simulink model "cordicModelComposer"  (R2021a)
settings: Solver=VariableStepAuto  StartTime=0.0  StopTime=50  RelTol=1e-3
undefined symbols (not defined in the file or in its folder): A, N
libraries: hdlBasic x26, hdlDSPIP x2, xbsIndex_r4 x1, JTAGRuntimeCosim_r4 x1
settings Model: Creator=Heather  LastModifiedBy=kv25
settings DebuggingCC: UnconnectedInputMsg=none  UnconnectedOutputMsg=none  UnconnectedLineMsg=none
settings ModelReferenceCC: EnableRefExpFcnMdlSchedulingChecks=off
settings RTWCC: Description=Generic Real-Time Target  DLArmComputeVersion=20.02.1

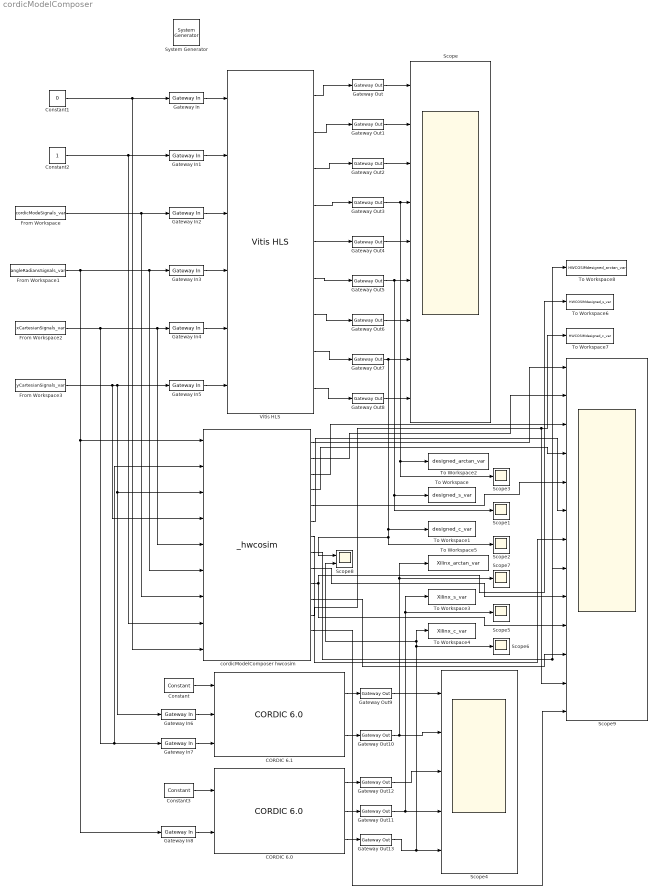
== system cordicModelComposer ==
  " System Generator" : xbsIndex_r4/ System Generator  Tag=genX  xilinxfamily=zynq  part=xc7z020  speed=-1  package=clg484  synthesis_tool=Vivado  clock_wrapper=Clock Enables  directory=./netlist369  proj_type=Vivado  Synth_file=Vivado Synthesis Defaults  Impl_file=Vivado Implementation Defaults  testbench=off  simulink_period=1  sysclk_period=10  dcm_input_clock_period=10  incr_netlist=off  trim_vbits=Everywhere in SubSystem  dbl_ovrd=According to Block Masks  core_generation=According to Block Masks  run_coregen=off  deprecated_control=off  eval_field=0  block_type=sysgen
  CORDIC 6.0 : hdlDSPIP/CORDIC 6.0   functional_selection=Sin_and_Cos  architectural_configuration=Parallel  pipelining_mode=Maximum  data_format=SignedFraction  phase_format=Radians  input_width=16  output_width=16  round_mode=Truncate  iterations=20  precision=0  compensation_scaling=No_Scale_Compensation  coarse_rotation=on  aclken=off  aresetn=off  out_tready=off  cartesian_has_tuser=off  cartesian_has_tlast=off  cartesian_tuser_width=1  phase_has_tuser=off  phase_has_tlast=off  phase_tuser_width=1  out_tlast_behv=Null  flow_control=NonBlocking  optimize_goal=Resources  trim_axipin_name=on  simulation_type=hybrid_sim  simulation_model=sysgen:cordic_v6_0  data_path_portlist={'s_axis_cartesian_tdata_imag', 's_axis_cartesian_tdata_real', 's_axis_phase_tdata_phase', 'm_axis_dout_tdata_imag', 'm_axis_dout_tdata_real', 'm_axis_dout_tdata_phase','m_axis_dout_tdata'}  ip_name=CORDIC  ip_version=6.0  dsptool_ready=true  ipcore_usecache=true  ipcore_useipmodelcache=true  wrapper_available=true  port_translation_map={ 'aclken' => 'en', 'aresetn' => 'rst' }  XmcBlockStatus=1  maskContainerNames=group15  block_type=cordic_v6_0  block_config=sysgen:rodinimport_config  block_width=800
  CORDIC 6.1 : hdlDSPIP/CORDIC 6.0   functional_selection=Arc_Tan  architectural_configuration=Parallel  pipelining_mode=Maximum  data_format=SignedFraction  phase_format=Radians  input_width=16  output_width=16  round_mode=Truncate  iterations=0  precision=0  compensation_scaling=No_Scale_Compensation  coarse_rotation=on  aclken=off  aresetn=off  out_tready=off  cartesian_has_tuser=off  cartesian_has_tlast=off  cartesian_tuser_width=1  phase_has_tuser=off  phase_has_tlast=off  phase_tuser_width=1  out_tlast_behv=Null  flow_control=NonBlocking  optimize_goal=Resources  trim_axipin_name=on  simulation_type=hybrid_sim  simulation_model=sysgen:cordic_v6_0  data_path_portlist={'s_axis_cartesian_tdata_imag', 's_axis_cartesian_tdata_real', 's_axis_phase_tdata_phase', 'm_axis_dout_tdata_imag', 'm_axis_dout_tdata_real', 'm_axis_dout_tdata_phase','m_axis_dout_tdata'}  ip_name=CORDIC  ip_version=6.0  dsptool_ready=true  ipcore_usecache=true  ipcore_useipmodelcache=true  wrapper_available=true  port_translation_map={ 'aclken' => 'en', 'aresetn' => 'rst' }  XmcBlockStatus=1  maskContainerNames=group15  block_type=cordic_v6_0  block_config=sysgen:rodinimport_config  block_width=800
  Constant : hdlBasic/Constant  const=1.0  gui_display_data_type=Boolean  arith_type=Boolean  n_bits=16  bin_pt=14  preci_type=Single  exp_width=8  frac_width=24  explicit_period=off  period=1  XmcBlockStatus=1  maskContainerNames=tabcontainer1  block_type=constant  block_config=sysgen:Constant_config
  Constant1 : Constant  Value=0
  Constant2 : Constant
  Constant3 : hdlBasic/Constant  const=1.0  gui_display_data_type=Boolean  arith_type=Boolean  n_bits=16  bin_pt=14  preci_type=Single  exp_width=8  frac_width=24  explicit_period=off  period=1  XmcBlockStatus=1  maskContainerNames=tabcontainer1  block_type=constant  block_config=sysgen:Constant_config
  From Workspace : FromWorkspace  VariableName=cordicModeSignals_var
  From Workspace1 : FromWorkspace  VariableName=angleRadiansSignals_var
  From Workspace2 : FromWorkspace  VariableName=xCartesianSignals_var
  From Workspace3 : FromWorkspace  VariableName=yCartesianSignals_var
  Gateway In : hdlBasic/Gateway In  gui_display_data_type=Boolean  arith_type=Boolean  n_bits=16  bin_pt=14  preci_type=Single  exp_width=8  frac_width=24  rows=1  columns=1  quantization="Round  (unbiased: +/- Inf)"  overflow=Saturate  period=1  UseAsADC=off  ADCChannel='1'  interface=None  automatic_assignment=on  address_offset=hex2dec('00')  intf_name=''  intf_description=''  default_value=0  timing_constraint=None  locs_specified=off  LOCs={}  io_standard={}  inherit_from_input=off  hdl_port=on  XmcBlockStatus=1  maskContainerNames=group4  block_type=gatewayin  block_config=sysgen:gateway_in_config  block_width_w=590  block_height_w=620  block_width=640  block_height=850
  Gateway In1 : hdlBasic/Gateway In  gui_display_data_type=Boolean  arith_type=Boolean  n_bits=16  bin_pt=3  preci_type=Single  exp_width=8  frac_width=24  rows=1  columns=1  quantization="Round  (unbiased: +/- Inf)"  overflow=Saturate  period=1  UseAsADC=off  ADCChannel='1'  interface=None  automatic_assignment=on  address_offset=hex2dec('00')  intf_name=''  intf_description=''  default_value=0  timing_constraint=None  locs_specified=off  LOCs={}  io_standard={}  inherit_from_input=off  hdl_port=on  XmcBlockStatus=1  maskContainerNames=group4  block_type=gatewayin  block_config=sysgen:gateway_in_config  block_width_w=590  block_height_w=620  block_width=640  block_height=850
  Gateway In2 : hdlBasic/Gateway In  gui_display_data_type=Boolean  arith_type=Boolean  n_bits=16  bin_pt=3  preci_type=Single  exp_width=8  frac_width=24  rows=1  columns=1  quantization="Round  (unbiased: +/- Inf)"  overflow=Saturate  period=1  UseAsADC=off  ADCChannel='1'  interface=None  automatic_assignment=on  address_offset=hex2dec('00')  intf_name=''  intf_description=''  default_value=0  timing_constraint=None  locs_specified=off  LOCs={}  io_standard={}  inherit_from_input=off  hdl_port=on  XmcBlockStatus=1  maskContainerNames=group4  block_type=gatewayin  block_config=sysgen:gateway_in_config  block_width_w=590  block_height_w=620  block_width=640  block_height=850
  Gateway In{3..5,8} (4 alike) : hdlBasic/Gateway In  gui_display_data_type=Fixed-point  arith_type=Signed (2's comp)  n_bits=16  bin_pt=13  preci_type=Single  exp_width=8  frac_width=24  rows=1  columns=1  quantization="Round  (unbiased: +/- Inf)"  overflow=Saturate  period=1  UseAsADC=off  ADCChannel='1'  interface=None  automatic_assignment=on  address_offset=hex2dec('00')  intf_name=''  intf_description=''  default_value=0  timing_constraint=None  locs_specified=off  LOCs={}  io_standard={}  inherit_from_input=off  hdl_port=on  XmcBlockStatus=1  maskContainerNames=group4  block_type=gatewayin  block_config=sysgen:gateway_in_config  block_width_w=590  block_height_w=620  block_width=640  block_height=850
  Gateway In6 : hdlBasic/Gateway In  gui_display_data_type=Fixed-point  arith_type=Signed (2's comp)  n_bits=16  bin_pt=14  preci_type=Single  exp_width=8  frac_width=24  rows=1  columns=1  quantization="Round  (unbiased: +/- Inf)"  overflow=Saturate  period=1  UseAsADC=off  ADCChannel='1'  interface=None  automatic_assignment=on  address_offset=hex2dec('00')  intf_name=''  intf_description=''  default_value=0  timing_constraint=None  locs_specified=off  LOCs={}  io_standard={}  inherit_from_input=off  hdl_port=on  XmcBlockStatus=1  maskContainerNames=group4  block_type=gatewayin  block_config=sysgen:gateway_in_config  block_width_w=590  block_height_w=620  block_width=640  block_height=850
  Gateway In7 : hdlBasic/Gateway In  gui_display_data_type=Fixed-point  arith_type=Signed (2's comp)  n_bits=16  bin_pt=14  preci_type=Single  exp_width=8  frac_width=24  rows=1  columns=1  quantization="Round  (unbiased: +/- Inf)"  overflow=Saturate  period=1  UseAsADC=off  ADCChannel='1'  interface=None  automatic_assignment=on  address_offset=hex2dec('00')  intf_name=''  intf_description=''  default_value=0  timing_constraint=None  locs_specified=off  LOCs={}  io_standard={}  inherit_from_input=off  hdl_port=on  XmcBlockStatus=1  maskContainerNames=group4  block_type=gatewayin  block_config=sysgen:gateway_in_config  block_width_w=590  block_height_w=620  block_width=640  block_height=850
  Gateway Out{,1..13} (14 alike) : hdlBasic/Gateway Out  inherit_from_input=off  hdl_port=on  rows=1  columns=1  UseAsDAC=off  DACChannel='1'  interface=None  automatic_assignment=on  address_offset=hex2dec('00')  intf_name=''  intf_description=''  timing_constraint=None  locs_specified=off  LOCs={}  io_standard={}  XmcBlockStatus=1  maskContainerNames=group4  block_type=gatewayout  block_config=sysgen:gateway_out_config  block_width_w=590  block_height_w=620  block_width=620  block_height=750
  Scope : Scope  NumInputPorts=9
  Scope{1..3,5..7} (6 alike) : Scope
  Scope4 : Scope  NumInputPorts=5
  Scope8 : Scope  NumInputPorts=2
  Scope9 : Scope  NumInputPorts=13
  To Workspace : ToWorkspace  VariableName=designed_s_var  SaveFormat=Timeseries  SampleTime=-1
  To Workspace1 : ToWorkspace  VariableName=designed_c_var  SaveFormat=Timeseries  SampleTime=-1
  To Workspace2 : ToWorkspace  VariableName=designed_arctan_var  SaveFormat=Timeseries  SampleTime=-1
  To Workspace3 : ToWorkspace  VariableName=Xilinx_s_var  SaveFormat=Timeseries  SampleTime=-1
  To Workspace4 : ToWorkspace  VariableName=Xilinx_c_var  SaveFormat=Timeseries  SampleTime=-1
  To Workspace5 : ToWorkspace  VariableName=Xilinx_arctan_var  SaveFormat=Timeseries  SampleTime=-1
  To Workspace6 : ToWorkspace  VariableName=HWCOSIMdesigned_s_var  SaveFormat=Timeseries  SampleTime=-1
  To Workspace7 : ToWorkspace  VariableName=HWCOSIMdesigned_c_var  SaveFormat=Timeseries  SampleTime=-1
  To Workspace8 : ToWorkspace  VariableName=HWCOSIMdesigned_arctan_var  SaveFormat=Timeseries  SampleTime=-1
  Vitis HLS : hdlBasic/Vitis HLS  anytable='C:\ELEC522\venaik\Project4\Vitis_HLS\cordic\solution1'  fast_sim=on  display_datatype=off  rate_propagation_method=Simulink system period  model_file_path=''  latency=1  block_type=vitis_hls
      settings: infoedit=This block allows including C,C++ and SystemC source files in System Generator for DSP designs.
  cordicModelComposer hwcosim : JTAGRuntimeCosim_r4/_hwcosim  clkSrc=Single Stepped  hasCombinationalPath=on  bitfileName=C:\ELEC522\venaik\Project4\Vitis_MC\netlist369\cordicmodelcomposer.bit  skipConfig=off  dispPartInfo=off  useZynqReconfigScript=on  cable=Auto Detect  speed=N/A  cablePort=N/A  cableLocation=Local  shareCable=off  xmp=[]  software_settings=[]  design_xtable=|  binDir=[]  engineDll=JTAGCosimEngine.dll  cableWaitTime=10  bscanPos=-1  IRLengths=[]  useWaitBox=1  hasBufgmux=on  Scheme=Cosim  useCmdProc=1  hasProc=0  useImpact=0  printLogFile=0  userChain=2  XmcBlockStatus=0  maskContainerNames=tabcontainer1  block_type=jtagcosim  block_config=Sysgen:hwcosim_block_config
      | {
      |     'clkWrapper' => 'cordicmodelcomposer',
      |     'burstMode' => false,
      |     'burstFifoDepth' => '1024',
      |     'shared_memories' => {},
      |     'clocksGcd' => 1,
      |     'device' => {
      |       'family' => 'zynq',
      |       'part' => 'xc7z020',
      |       'package' => 'clg484',
      |       'speed' => '-1',
      |     },
      |     'ports' => {
      |       'gateway_in8' => {
      |         'direction' => 'in',
      |         'width' => 16,
      |         'name' => 'gateway_in8',
      |         'period' => 1,
      |         'icon_text' => 'Gateway In8',
      |         'type' => 'Fix_16_13',
      |         'arithmetic_type' => 'xlSigned',
      |         'dat_file' => 'cordicmodelcomposer_gateway_in8.dat',
      |         'bin_pt' => 13,
      |         'addr_offset' => 0,
      |         'bd_port_index' => 0,
      |       },
      |       'gateway_in7' => {
      |         'direction' => 'in',
      |         'width' => 16,
      |         'name' => 'gateway_in7',
      |         'period' => 1,
      |         'icon_text' => 'Gateway In7',
      |         'type' => 'Fix_16_14',
      |         'arithmetic_type' => 'xlSigned',
      |         'dat_file' => 'cordicmodelcomposer_gateway_in7.dat',
      |         'bin_pt' => 14,
      |         'addr_offset' => 4,
      |         'bd_port_index' => 1,
      |       },
      |       'gateway_in6' => {
      |         'direction' => 'in',
      |         'width' => 16,
      |         'name' => 'gateway_in6',
      |         'period' => 1,
      |         'icon_text' => 'Gateway In6',
      |         'type' => 'Fix_16_14',
      |         'arithmetic_type' => 'xlSigned',
      |         'dat_file' => 'cordicmodelcomposer_gateway_in6.dat',
      |         'bin_pt' => 14,
      |         'addr_offset' => 8,
      |         'bd_port_index' => 2,
      |       },
      |       'gateway_in5' => {
      |         'direction' => 'in',
      |         'width' => 16,
      |         'name' => 'gateway_in5',
      |         'period' => 1,
      |         'icon_text' => 'Gateway In5',
      |         'type' => 'Fix_16_13',
      |         'arithmetic_type' => 'xlSigned',
      |         'dat_file' => 'cordicmodelcomposer_gateway_in5.dat',
      |         'bin_pt' => 13,
      |         'addr_offset' => 12,
      |         'bd_port_index' => 3,
      |       },
      |       'gateway_in4' => {
      |         'direction' => 'in',
      |         'width' => 16,
      |         'name' => 'gateway_in4',
      |         'period' => 1,
      |         'icon_text' => 'Gateway In4',
      |         'type' => 'Fix_16_13',
      |         'arithmetic_type' => 'xlSigned',
      |         'dat_file' => 'cordicmodelcomposer_gateway_in4.dat',
      |         'bin_pt' => 13,
      |         'addr_offset' => 16,
      |         'bd_port_index' => 4,
      |       },
      |       'gateway_in3' => {
      |         'direction' => 'in',
      |         'width' => 16,
      |         'name' => 'gateway_in3',
      |         'period' => 1,
      |         'icon_text' => 'Gateway In3',
      |         'type' => 'Fix_16_13',
      |         'arithmetic_type' => 'xlSigned',
      |         'dat_file' => 'cordicmodelcomposer_gateway_in3.dat',
      |         'bin_pt' => 13,
      |         'addr_offset' => 20,
      |         'bd_port_index' => 5,
      |       },
      |       'gateway_in2' => {
      |         'direction' => 'in',
      |         'width' => 1,
      |         'name' => 'gateway_in2',
      |         'period' => 1,
      |         'icon_text' => 'Gateway In2',
      |         'type' => 'Bool',
      |         'arithmetic_type' => 'xlUnsigned',
      |         'dat_file' => 'cordicmodelcomposer_gateway_in2.dat',
      |         'bin_pt' => 0,
      |         'addr_offset' => 24,
      |         'bd_port_index' => 6,
      |       },
      |       'gateway_in1' => {
      |         'direction' => 'in',
      |         'width' => 1,
      |         'name' => 'gateway_in1',
      |         'period' => 1,
      |         'icon_text' => 'Gateway In1',
      |         'type' => 'Bool',
      |         'arithmetic_type' => 'xlUnsigned',
      |         'dat_file' => 'cordicmodelcomposer_gateway_in1.dat',
      |         'bin_pt' => 0,
      |         'addr_offset' => 28,
      |         'bd_port_index' => 7,
      |       },
      |       'gateway_in' => {
      |         'direction' => 'in',
      |         'width' => 1,
      |         'name' => 'gateway_in',
      |         'period' => 1,
      |         'icon_text' => 'Gateway In',
      |         'type' => 'Bool',
      |         'arithmetic_type' => 'xlUnsigned',
      |         'dat_file' => 'cordicmodelcomposer_gateway_in.dat',
      |         'bin_pt' => 0,
      |         'addr_offset' => 32,
      |         'bd_port_index' => 8,
      |       },
      |       'gateway_out' => {
      |         'direction' => 'out',
      |         'width' => 1,
      |         'name' => 'gateway_out',
      |         'period' => 1,
      |         'icon_text' => 'Gateway Out',
      |         'type' => 'Bool',
      |         'arithmetic_type' => 'xlUnsigned',
      |         'dat_file' => 'cordicmodelcomposer_gateway_out.dat',
      |         'bin_pt' => 0,
      |         'addr_offset' => 36,
      |         'bd_port_index' => 0,
      |       },
      |       'gateway_out1' => {
      |         'direction' => 'out',
      |         'width' => 1,
      |         'name' => 'gateway_out1',
      |         'period' => 1,
      |         'icon_text' => 'Gateway Out1',
      |         'type' => 'Bool',
      |         'arithmetic_type' => 'xlUnsigned',
      |         'dat_file' => 'cordicmodelcomposer_gateway_out1.dat',
      |         'bin_pt' => 0,
      |         'addr_offset' => 40,
      |         'bd_port_index' => 1,
      |       },
      |       'gateway_out10' => {
      |         'direction' => 'out',
      |         'width' => 16,
      |         'name' => 'gateway_out10',
      |         'period' => 1,
      |         'icon_text' => 'Gateway Out10',
      |         'type' => 'Fix_16_13',
      |         'arithmetic_type' => 'xlSigned',
      |         'dat_file' => 'cordicmodelcomposer_gateway_out10.dat',
      |         'bin_pt' => 13,
      |         'addr_offset' => 44,
      |         'bd_port_index' => 2,
      |       },
      |       'gateway_out11' => {
      |         'direction' => 'out',
      |         'width' => 16,
      |         'name' => 'gateway_out11',
      |         'period' => 1,
      |         'icon_text' => 'Gateway Out11',
      |         'type' => 'Fix_16_14',
      |         'arithmetic_type' => 'xlSigned',
      |         'dat_file' => 'cordicmodelcomposer_gateway_out11.dat',
      |         'bin_pt' => 14,
      |         'addr_offset' => 48,
      |         'bd_port_index' => 3,
      |       },
      |       'gateway_out12' => {
      |         'direction' => 'out',
      |         'width' => 1,
      |         'name' => 'gateway_out12',
      |         'period' => 1,
      |         'icon_text' => 'Gateway Out12',
      |         'type' => 'Bool',
      |         'arithmetic_type' => 'xlUnsigned',
      |         'dat_file' => 'cordicmodelcomposer_gateway_out12.dat',
      |         'bin_pt' => 0,
      |         'addr_offset' => 52,
      |         'bd_port_index' => 4,
      |       },
      |       'gateway_out13' => {
      |         'direction' => 'out',
      |         'width' => 16,
      |         'name' => 'gateway_out13',
      |         'period' => 1,
      |         'icon_text' => 'Gateway Out13',
      |         'type' => 'Fix_16_14',
      |         'arithmetic_type' => 'xlSigned',
      |         'dat_file' => 'cordicmodelcomposer_gateway_out13.dat',
      |         'bin_pt' => 14,
      |         'addr_offset' => 56,
      |         'bd_port_index' => 5,
      |       },
      |       'gateway_out2' => {
      |         'direction' => 'out',
      |         'width' => 1,
      |         'name' => 'gateway_out2',
      |         'period' => 1,
      |         'icon_text' => 'Gateway Out2',
      |         'type' => 'Bool',
      |         'arithmetic_type' => 'xlUnsigned',
      |         'dat_file' => 'cordicmodelcomposer_gateway_out2.dat',
      |         'bin_pt' => 0,
      |         'addr_offset' => 60,
      |         'bd_port_index' => 6,
      |       },
      |       'gateway_out3' => {
      |         'direction' => 'out',
      |         'width' => 16,
      |         'name' => 'gateway_out3',
      |         'period' => 1,
      |         'icon_text' => 'Gateway Out3',
      |         'type' => 'Fix_16_13',
      |         'arithmetic_type' => 'xlSigned',
      |         'dat_file' => 'cordicmodelcomposer_gateway_out3.dat',
      |         'bin_pt' => 13,
      |         'addr_offset' => 64,
      |         'bd_port_index' => 7,
      |       },
      |       'gateway_out4' => {
      |         'direction' => 'out',
      |         'width' => 1,
      |         'name' => 'gateway_out4',
      |         'period' => 1,
      |         'icon_text' => 'Gateway Out4',
      |         'type' => 'Bool',
      |         'arithmetic_type' => 'xlUnsigned',
      |         'dat_file' => 'cordicmodelcomposer_gateway_out4.dat',
      |         'bin_pt' => 0,
      |         'addr_offset' => 68,
      |         'bd_port_index' => 8,
      |       },
      |       'gateway_out5' => {
      |         'direction' => 'out',
      |         'width' => 16,
      |         'name' => 'gateway_out5',
      |         'period' => 1,
      |         'icon_text' => 'Gateway Out5',
      |         'type' => 'Fix_16_13',
      |         'arithmetic_type' => 'xlSigned',
      |         'dat_file' => 'cordicmodelcomposer_gateway_out5.dat',
      |         'bin_pt' => 13,
      |         'addr_offset' => 72,
      |         'bd_port_index' => 9,
      |       },
      |       'gateway_out6' => {
      |         'direction' => 'out',
      |         'width' => 1,
      |         'name' => 'gateway_out6',
      |         'period' => 1,
      |         'icon_text' => 'Gateway Out6',
      |         'type' => 'Bool',
      |         'arithmetic_type' => 'xlUnsigned',
      |         'dat_file' => 'cordicmodelcomposer_gateway_out6.dat',
      |         'bin_pt' => 0,
      |         'addr_offset' => 76,
      |         'bd_port_index' => 10,
      |       },
      |       'gateway_out7' => {
      |         'direction' => 'out',
      |         'width' => 16,
      |         'name' => 'gateway_out7',
      |         'period' => 1,
      |         'icon_text' => 'Gateway Out7',
      |         'type' => 'Fix_16_13',
      |         'arithmetic_type' => 'xlSigned',
      |         'dat_file' => 'cordicmodelcomposer_gateway_out7.dat',
      |         'bin_pt' => 13,
      |         'addr_offset' => 80,
      |         'bd_port_index' => 11,
      |       },
      |       'gateway_out8' => {
      |         'direction' => 'out',
      |         'width' => 1,
      |         'name' => 'gateway_out8',
      |         'period' => 1,
      |         'icon_text' => 'Gateway Out8',
      |         'type' => 'Bool',
      |         'arithmetic_type' => 'xlUnsigned',
      |         'dat_file' => 'cordicmodelcomposer_gateway_out8.dat',
      |         'bin_pt' => 0,
      |         'addr_offset' => 84,
      |         'bd_port_index' => 12,
      |       },
      |       'gateway_out9' => {
      |         'direction' => 'out',
      |         'width' => 1,
      |         'name' => 'gateway_out9',
      |         'period' => 1,
      |         'icon_text' => 'Gateway Out9',
      |         'type' => 'Bool',
      |         'arithmetic_type' => 'xlUnsigned',
      |         'dat_file' => 'cordicmodelcomposer_gateway_out9.dat',
      |         'bin_pt' => 0,
      |         'addr_offset' => 88,
      |         'bd_port_index' => 13,
      |       },
      |     },
      |   }
  wires:
  Constant2/1 -> cordicModelComposer hwcosim/8, Gateway In1/1
  Gateway In1/1 -> Vitis HLS/2
  Gateway In/1 -> Vitis HLS/1
  Constant1/1 -> cordicModelComposer hwcosim/9, Gateway In/1
  Vitis HLS/1 -> Gateway Out/1
  Vitis HLS/2 -> Gateway Out1/1
  Gateway Out/1 -> Scope/1
  Gateway Out1/1 -> Scope/2
  Gateway Out2/1 -> Scope/3
  Gateway Out4/1 -> Scope/5
  Gateway Out5/1 -> Scope/6, To Workspace/1, Scope1/1
  Gateway Out6/1 -> Scope/7
  Gateway Out7/1 -> Scope/8, Scope8/1, Scope2/1, To Workspace1/1
  Gateway Out8/1 -> Scope/9
  From Workspace/1 -> cordicModelComposer hwcosim/7, Gateway In2/1
  Gateway In3/1 -> Vitis HLS/4
  From Workspace1/1 -> Gateway In8/1, cordicModelComposer hwcosim/1, cordicModelComposer hwcosim/6, Gateway In3/1
  Gateway In2/1 -> Vitis HLS/3
  From Workspace3/1 -> cordicModelComposer hwcosim/4, Gateway In6/1, cordicModelComposer hwcosim/3, Gateway In5/1
  From Workspace2/1 -> cordicModelComposer hwcosim/2, Gateway In7/1, cordicModelComposer hwcosim/5, Gateway In4/1
  Gateway In5/1 -> Vitis HLS/6
  Gateway In4/1 -> Vitis HLS/5
  Gateway Out3/1 -> To Workspace2/1, Scope3/1, Scope/4
  CORDIC 6.1/1 -> Gateway Out9/1
  CORDIC 6.1/2 -> Gateway Out10/1
  CORDIC 6.0/1 -> Gateway Out12/1
  CORDIC 6.0/2 -> Gateway Out11/1
  CORDIC 6.0/3 -> Gateway Out13/1
  Gateway Out9/1 -> Scope4/1
  Gateway Out10/1 -> Scope7/1, To Workspace5/1, Scope4/2
  Gateway Out12/1 -> Scope4/3
  Gateway Out11/1 -> Scope5/1, To Workspace3/1, Scope4/4
  Gateway Out13/1 -> Scope4/5, Scope6/1, Scope8/2, To Workspace4/1
  Constant/1 -> CORDIC 6.1/1
  Constant3/1 -> CORDIC 6.0/1
  Gateway In6/1 -> CORDIC 6.1/2
  Gateway In8/1 -> CORDIC 6.0/2
  Gateway In7/1 -> CORDIC 6.1/3
  Vitis HLS/3 -> Gateway Out2/1
  Vitis HLS/4 -> Gateway Out3/1
  Vitis HLS/5 -> Gateway Out4/1
  Vitis HLS/6 -> Gateway Out5/1
  Vitis HLS/7 -> Gateway Out6/1
  Vitis HLS/8 -> Gateway Out7/1
  Vitis HLS/9 -> Gateway Out8/1
  cordicModelComposer hwcosim/1 -> Scope9/1
  cordicModelComposer hwcosim/2 -> Scope9/2
  cordicModelComposer hwcosim/3 -> Scope9/3
  cordicModelComposer hwcosim/4 -> Scope9/4
  cordicModelComposer hwcosim/5 -> Scope9/5
  cordicModelComposer hwcosim/6 -> Scope9/6
  cordicModelComposer hwcosim/7 -> Scope9/7
  cordicModelComposer hwcosim/8 -> To Workspace8/1, Scope9/8
  cordicModelComposer hwcosim/9 -> Scope9/9
  cordicModelComposer hwcosim/10 -> To Workspace6/1, Scope9/10
  cordicModelComposer hwcosim/11 -> Scope9/11
  cordicModelComposer hwcosim/12 -> To Workspace7/1, Scope9/12
  cordicModelComposer hwcosim/13 -> Scope9/13
